simulink model "STEVE_Simulation"  (R2024b)
settings: Solver=ode4  StartTime=0.0  StopTime=60*1  FixedStep=0.001  RelTol=1e-3  EnableMultiTasking=on
values from neighbouring files (symbols this model uses):
  alphaValues = unique(data.Alpha)    [initialize_aeroData.m]    (also in initialize_parameters.m; lookup_data.mat = [0 2 4])
  CL_grid = nan(length(alphaValues), length(machValues))    [initialize_aeroData.m]    (also in initialize_parameters.m; lookup_data.mat = [0 0.430502365793 0.859237162153 0 0.432754592992 0.86375537)
  machValues = unique(data.Mach)    [initialize_aeroData.m]    (also in initialize_parameters.m; lookup_data.mat = [0.01 0.02 0.03 0.04 0.05 0.06 0.07 0.08 0.09 0.1 0.11 0.12 )
  max_thrust = 50    [initialize_parameters.m]
libraries: simulink x2, aerolibwind2 x1, aerolibatmos2 x1, simulink_extras x1, slpidlib x1, aerolibnav x1, aerolibasang x1, aerolibactuator x1
settings Model: ExtModeTrigDuration=2  Creator=jonno  LastModifiedBy=jonno
settings SolverCC: AutoInsertRateTranBlk=on
settings RTWCC: BuildConfiguration=Faster Runs

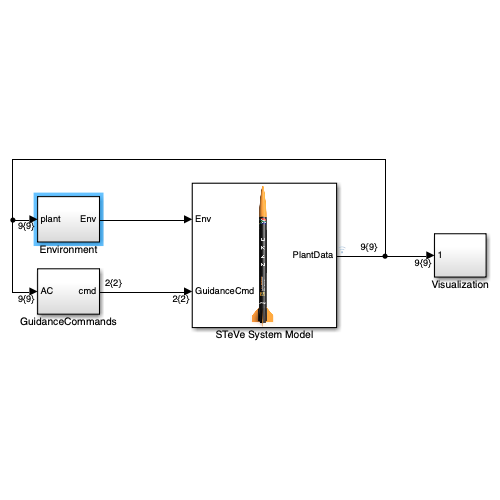
[thumbnail: Simulink's stored preview of the top-level diagram]
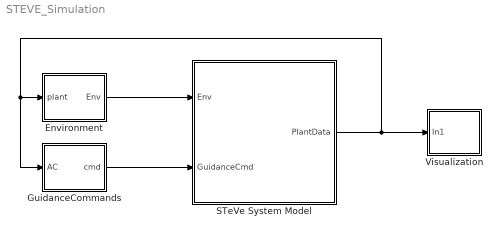
== system STEVE_Simulation ==
  Environment : Subsystem
  GuidanceCommands : Subsystem
  STeVe System Model : Subsystem
      mask Display: image('steve.png', [65 - (50 * (187 / 1041)), 0, 140 * (187 / 1041), 140])
  Visualization : Subsystem
  wires:
  GuidanceCommands/1(cmd) -> STeVe System Model/2(GuidanceCmd)
  Environment/1(Env) -> STeVe System Model/1(Env)
  STeVe System Model/1(PlantData) -> GuidanceCommands/1(AC), Environment/1(plant), Visualization/1(In1)

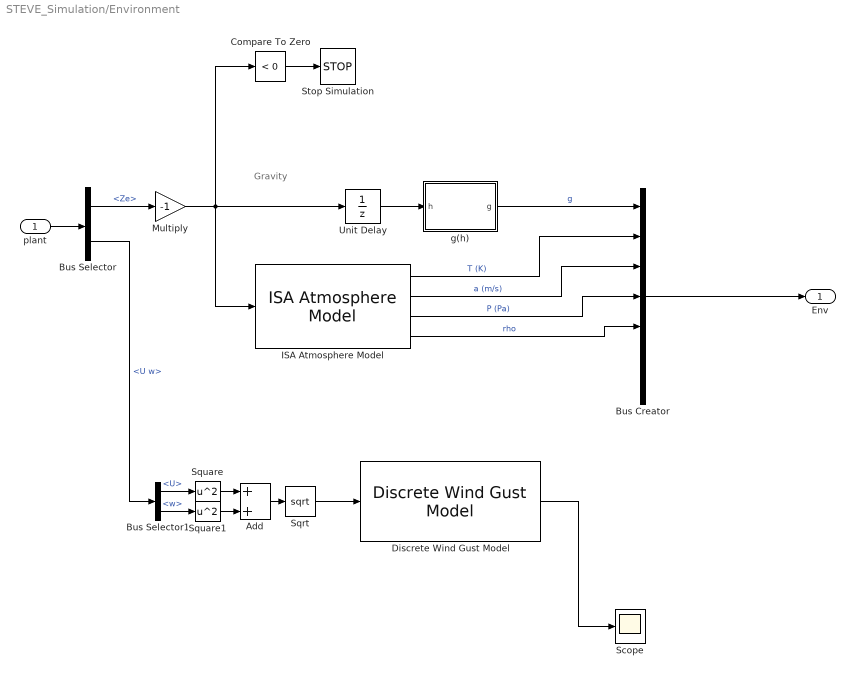
== system STEVE_Simulation/Environment ==
  note: Gravity
  plant : Inport
  Add : Sum
  Bus Creator : BusCreator  Inputs=7
  Bus Selector : BusSelector  OutputSignals=XeZe.Ze,U w
  Bus Selector1 : BusSelector  OutputSignals=U,w
  Compare To Zero : simulink/Logic and Bit Operations/Compare To Zero  relop=<  OutDataTypeStr=boolean
  Discrete Wind Gust Model : aerolibwind2/Discrete Wind Gust Model  units=Metric (MKS)  Gx=on  Gy=off  Gz=on  t_0=5  d_m=[120 120 80]  v_m=[3.5 3.5 3.0]
  ISA Atmosphere Model : aerolibatmos2/ISA Atmosphere Model  useExtended=on  action=Warning  custom=off  viscosityOut=off  g=9.80665  gamma=1.4  R=287.0531  L=0.0065  h_trop=11000  h_strat=20000  rho0=1.225  P0=101325  T0=288.15  h0=0  S=110.4  Tref=273.15  muref=1.716e-5
  Multiply : Gain  Gain=-1
  Scope : Scope
  Sqrt : Sqrt
  Square : Math  Operator=square
  Square1 : Math  Operator=square
  Stop Simulation : Stop
  Unit Delay : UnitDelay  SampleTime=-1  HasFrameUpgradeWarning=on
  g(h) : MATLAB Function  TreatAsAtomicUnit=on
  Env : Outport
  wires:
  g(h)/1(g) -> Bus Creator/1  "g"
  plant/1 -> Bus Selector/1
  Bus Selector/1 -> Multiply/1  "<Ze>"
  Bus Creator/1 -> Env/1
  Unit Delay/1 -> g(h)/1(h)
  Compare To Zero/1 -> Stop Simulation/1
  Multiply/1 -> ISA Atmosphere Model/1, Unit Delay/1, Compare To Zero/1
  ISA Atmosphere Model/1 -> Bus Creator/2  "T (K)"
  ISA Atmosphere Model/2 -> Bus Creator/3  "a (m/s)"
  ISA Atmosphere Model/3 -> Bus Creator/4  "P (Pa)"
  ISA Atmosphere Model/4 -> Bus Creator/5  "rho"
  ? -> Bus Creator/6  "u_wind_body"
  ? -> Bus Creator/7  "w_wind_body"
  Bus Selector/2 -> Bus Selector1/1  "<U w>"
  Bus Selector1/1 -> Square/1  "<U>"
  Bus Selector1/2 -> Square1/1  "<w>"
  Square1/1 -> Add/2
  Square/1 -> Add/1
  Add/1 -> Sqrt/1
  Sqrt/1 -> Discrete Wind Gust Model/1
  Discrete Wind Gust Model/1 -> Scope/1

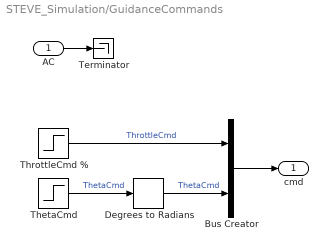
== system STEVE_Simulation/GuidanceCommands ==
  AC : Inport
  Bus Creator : BusCreator  Inputs=2
  Degrees to Radians : simulink_extras/Transformations/Degrees to Radians
  Terminator : Terminator
  ThetaCmd : Step  Before=90  After=170  SampleTime=0
  ThrottleCmd % : Step  Time=5  Before=100  After=0  SampleTime=0
  cmd : Outport
  wires:
  AC/1 -> Terminator/1
  ThrottleCmd %/1 -> Bus Creator/1  "ThrottleCmd"
  Bus Creator/1 -> cmd/1
  ThetaCmd/1 -> Degrees to Radians/1  "ThetaCmd"
  Degrees to Radians/1 -> Bus Creator/2  "ThetaCmd"

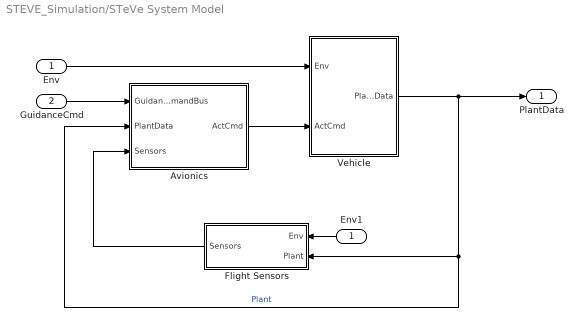
== system STEVE_Simulation/STeVe System Model ==
  Env : Inport
  GuidanceCmd : Inport  Port=2
  Avionics : Subsystem
  Env1 : InportShadow
  Flight Sensors : Subsystem
  Vehicle : Subsystem
  PlantData : Outport
  wires:
  Env/1 -> Vehicle/1(Env)
  Vehicle/1(PlantData) -> PlantData/1, Avionics/2(PlantData), Flight Sensors/2(Plant)  "Plant"
  Avionics/1(ActCmd) -> Vehicle/2(ActCmd)
  GuidanceCmd/1 -> Avionics/1(GuidanceCommandBus)
  Env1/1 -> Flight Sensors/1(Env)
  Flight Sensors/1(Sensors) -> Avionics/3(Sensors)

== system STEVE_Simulation/Visualization ==
  In1 : Inport
  Bus Selector : BusSelector  OutputSignals=XeZe
  Bus Selector1 : BusSelector  OutputSignals=Xe,Ze
  Compare To Zero : simulink/Logic and Bit Operations/Compare To Zero  relop=<  OutDataTypeStr=boolean
  Multiply : Gain  Gain=-1
  Stop Simulation : Stop
  XY Graph : Record  FileSettingsInternal="{\"entries\":[{\"content\":{\"excelSettings\":{\"content\":{},\"type\":\"Streamout.ExcelSettings\"}},\"type\":\"Streamout.FileSettingStorage\",\"uuid\":\"\"}],\"packageUris\":[\"http:\\/\\/schema.mathworks.com\\/mf0\\/streamout_blocks\\/R2020a\"],\"version\":\"1.0\"}"  Layout=[1 1]  SignalsInternal="{\"entries\":[{\"content\":{\"signals\":[{\"content\":{\"blockPath\":[],\"dimensions\":[1],\"domain\":\"\",\"lineColor\":\"#a2142f\",\"plots\":[ 1 ],\"port\":1,\"sid\":[\"\"],\"signalID\":1,\"signalName\":\"<Xe>\"},\"type\":\"RecordBlkView.Signal\",\"uuid\":\"\"},{\"content\":{\"blockPath\":[],\"dimensions\":[1],\"domain\":\"\",\"lineColor\":\"#139fff\",\"plots\":[ 1 ],\"port\":2,\"sid\":[\"\"],\"signalID\":2,\"signalName\":\"Multiply\"},\"type\":\"RecordBlkView.Signal\",\"uuid\":\"\"}]},\"type\":\"RecordBlkView.InputSignals\",\"uuid\":\"\"}],\"packageUris\":[\"http:\\/\\/schema.mathworks.com\\/mf0\\/streamout_blocks\\/R2020a\"],\"version\":\"1.0\"}"  VisualizationBindings="{\"xyplotplugin\":{\"info\":[{\"series\":[{\"bindingParametersList\":[{\"parameter\":\"X-Axis\",\"signalID\":1,\"signalName\":\"<Xe>\"},{\"parameter\":\"Y-Axis\",\"signalID\":2,\"signalName\":\"Multiply\"}],\"seriesID\":0}],\"subplotID\":1}]}}"  CompatibilityTag=XY
  wires:
  In1/1 -> Bus Selector/1
  Bus Selector/1 -> Bus Selector1/1  "<XeZe>"
  Bus Selector1/1 -> XY Graph/1  "<Xe>"
  Compare To Zero/1 -> Stop Simulation/1
  Bus Selector1/2 -> Multiply/1  "<Ze>"
  Multiply/1 -> Compare To Zero/1, XY Graph/2

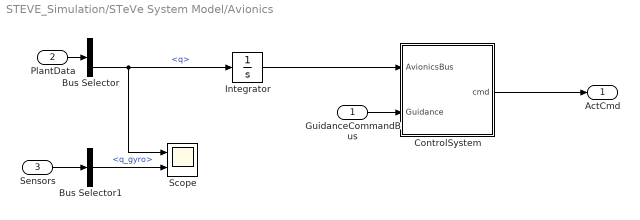
== system STEVE_Simulation/STeVe System Model/Avionics ==
  GuidanceCommandBus : Inport
  PlantData : Inport  Port=2
  Sensors : Inport  Port=3
  Bus Selector : BusSelector  OutputSignals=theta,q
  Bus Selector1 : BusSelector  OutputSignals=q_gyro
  ControlSystem : Subsystem
  Integrator : Integrator  InitialCondition=90*pi/180
  Scope : Scope  NumInputPorts=2
  ActCmd : Outport
  wires:
  PlantData/1 -> Bus Selector/1
  GuidanceCommandBus/1 -> ControlSystem/2(Guidance)
  ControlSystem/1(cmd) -> ActCmd/1
  Integrator/1 -> ControlSystem/1(AvionicsBus)
  Sensors/1 -> Bus Selector1/1
  Bus Selector/2 -> Scope/1, Integrator/1  "<q>"
  Bus Selector1/1 -> Scope/2  "<q_gyro>"

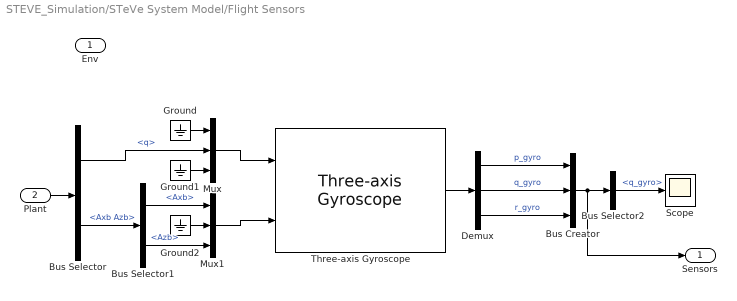
== system STEVE_Simulation/STeVe System Model/Flight Sensors ==
  Env : Inport
  Plant : Inport  Port=2
  Bus Creator : BusCreator  Inputs=3
  Bus Selector : BusSelector  OutputSignals=q,Axb Azb
  Bus Selector1 : BusSelector  OutputSignals=Axb,Azb
  Bus Selector2 : BusSelector  OutputSignals=q_gyro
  Demux : Demux  Outputs=3
  Ground : Ground
  Ground1 : Ground
  Ground2 : Ground
  Mux : Mux  Inputs=3
  Mux1 : Mux  Inputs=3
  Scope : Scope
  Three-axis Gyroscope : aerolibnav/Three-axis Gyroscope  dtype_g=on  w_g=190  z_g=0.707  g_sf_cc=[1 0 0; 0 1 0; 0 0 1]  g_bias=[0 0 0]  g_sen=[0 0 0]  g_Ts=0  g_rand=on  g_seeds=[23093 23094 23095]  g_pow=[0.0001 0.0001 0.0001]  g_sat="[-inf  -inf  -inf  inf inf inf]"
  Sensors : Outport
  wires:
  Plant/1 -> Bus Selector/1
  Mux/1 -> Three-axis Gyroscope/1
  Bus Selector/1 -> Mux/2  "<q>"
  Ground/1 -> Mux/1
  Ground1/1 -> Mux/3
  Mux1/1 -> Three-axis Gyroscope/2
  Bus Selector/2 -> Bus Selector1/1  "<Axb Azb>"
  Bus Selector1/1 -> Mux1/1  "<Axb>"
  Bus Selector1/2 -> Mux1/3  "<Azb>"
  Ground2/1 -> Mux1/2
  Three-axis Gyroscope/1 -> Demux/1
  Demux/1 -> Bus Creator/1  "p_gyro"
  Demux/2 -> Bus Creator/2  "q_gyro"
  Demux/3 -> Bus Creator/3  "r_gyro"
  Bus Creator/1 -> Sensors/1, Bus Selector2/1
  Bus Selector2/1 -> Scope/1  "<q_gyro>"

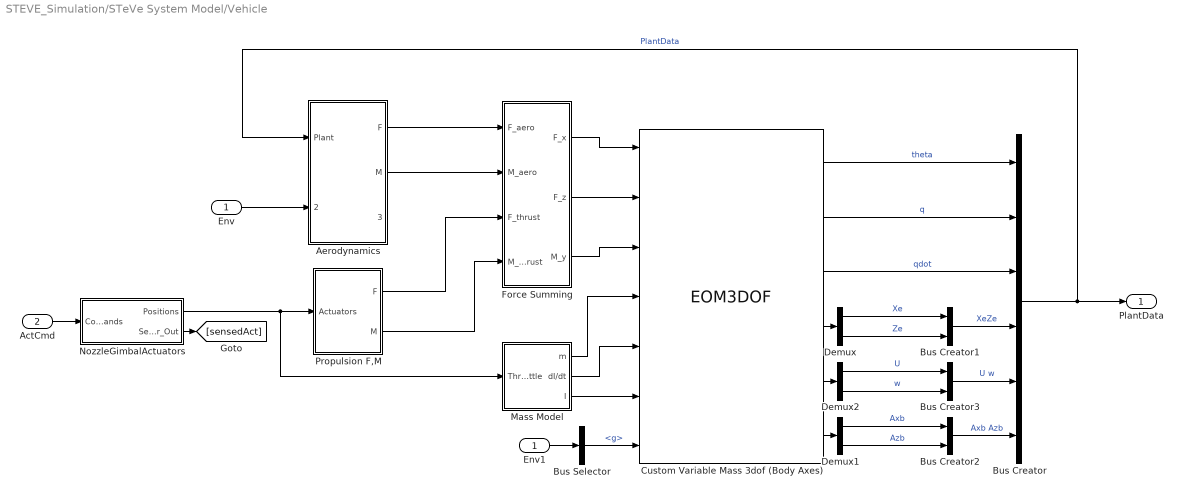
== system STEVE_Simulation/STeVe System Model/Vehicle ==
  Env : Inport
  ActCmd : Inport  Port=2
  Aerodynamics : Subsystem
  Bus Creator : BusCreator  Inputs=6
  Bus Creator1 : BusCreator  Inputs=2
  Bus Creator2 : BusCreator  Inputs=2
  Bus Creator3 : BusCreator  Inputs=2
  Bus Selector : BusSelector  OutputSignals=g
  Custom Variable Mass 3dof (Body Axes) : EOM3DOF  mtype=Custom Variable  v_ini=0  theta_ini=pi/2  g_in=External
  Demux : Demux  Outputs=2
  Demux1 : Demux  Outputs=2
  Demux2 : Demux  Outputs=2
  Env1 : InportShadow
  Force Summing : Subsystem
  Mass Model : Subsystem
  NozzleGimbalActuators : Subsystem
  Propulsion F,M : Subsystem
  PlantData : Outport
  wires:
  ActCmd/1 -> NozzleGimbalActuators/1(Commands)
  NozzleGimbalActuators/2(Sensor_Out) -> [sensedAct]
  NozzleGimbalActuators/1(Positions) -> Mass Model/1(Throttle), Propulsion F,M/1(Actuators)
  Force Summing/1(F_x) -> Custom Variable Mass 3dof (Body Axes)/1
  Force Summing/2(F_z) -> Custom Variable Mass 3dof (Body Axes)/2
  Aerodynamics/1(F) -> Force Summing/1(F_aero)
  Aerodynamics/2(M) -> Force Summing/2(M_aero)
  Propulsion F,M/1(F) -> Force Summing/3(F_thrust)
  Propulsion F,M/2(M) -> Force Summing/4(M_thrust)
  Force Summing/3(M_y) -> Custom Variable Mass 3dof (Body Axes)/3
  Mass Model/1(m) -> Custom Variable Mass 3dof (Body Axes)/4
  Mass Model/2(dI/dt) -> Custom Variable Mass 3dof (Body Axes)/5
  Mass Model/3(I) -> Custom Variable Mass 3dof (Body Axes)/6
  Custom Variable Mass 3dof (Body Axes)/1 -> Bus Creator/1  "theta"
  Custom Variable Mass 3dof (Body Axes)/2 -> Bus Creator/2  "q"
  Custom Variable Mass 3dof (Body Axes)/3 -> Bus Creator/3  "qdot"
  Bus Creator3/1 -> Bus Creator/5  "U w"
  Bus Creator2/1 -> Bus Creator/6  "Axb Azb"
  Bus Creator/1 -> Aerodynamics/1(Plant), PlantData/1  "PlantData"
  Bus Creator1/1 -> Bus Creator/4  "XeZe"
  Custom Variable Mass 3dof (Body Axes)/4 -> Demux/1
  Demux/1 -> Bus Creator1/1  "Xe"
  Demux/2 -> Bus Creator1/2  "Ze"
  Custom Variable Mass 3dof (Body Axes)/6 -> Demux1/1
  Demux1/1 -> Bus Creator2/1  "Axb"
  Demux1/2 -> Bus Creator2/2  "Azb"
  Custom Variable Mass 3dof (Body Axes)/5 -> Demux2/1
  Demux2/1 -> Bus Creator3/1  "U"
  Demux2/2 -> Bus Creator3/2  "w"
  Env/1 -> Aerodynamics/2(EnvData)
  Env1/1 -> Bus Selector/1
  Bus Selector/1 -> Custom Variable Mass 3dof (Body Axes)/7  "<g>"

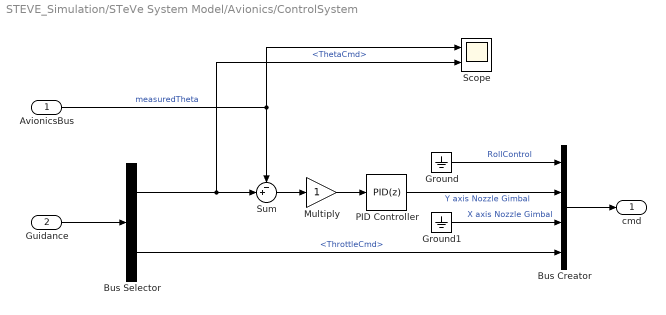
== system STEVE_Simulation/STeVe System Model/Avionics/ControlSystem ==
  AvionicsBus : Inport
  Guidance : Inport  Port=2
  Bus Creator : BusCreator  Inputs=4
  Bus Selector : BusSelector  OutputSignals=ThetaCmd,ThrottleCmd
  Ground : Ground
  Ground1 : Ground
  Multiply : Gain
  PID Controller : slpidlib/PID Controller  Controller=PID  Form=Parallel  TimeDomain=Discrete-time  UseExternalTs=off  SampleTime=-1  IntegratorMethod=Forward Euler  FilterMethod=Forward Euler  ControllerParametersSource=internal  P=1.9136005132319e-05  I=2.0107370615088e-06  UseKiTs=off  D=4.46649019604869e-05  UseExternalDerivativeSource=off  N=12.4167599537219  UseFilter=on  TunerSelectOption=Transfer Function Based (PID Tuner App)  InitialConditionSource=internal  InitialConditionForIntegrator=0  InitialConditionForFilter=0  DifferentiatorICPrevScaledInput=0  ExternalReset=none  TrackingMode=off  Kt=1  LimitOutput=off  SatLimitsSource=internal  UpperSaturationLimit=inf  LowerSaturationLimit=-inf  LinearizeAsGain=on  AntiWindupMode=none  Kb=1  LimitIntegrator=off  UpperIntegratorSaturationLimit=inf  LowerIntegratorSaturationLimit=-inf  POutMin=[]  POutMax=[]  IOutMin=[]  IOutMax=[]  DOutMin=[]  DOutMax=[]  NOutMin=[]  NOutMax=[]  SumOutMin=[]  SumOutMax=[]  SaturationOutMin=[]  SaturationOutMax=[]  PParamMin=[]  PParamMax=[]  IParamMin=[]  IParamMax=[]  DParamMin=[]  DParamMax=[]  NParamMin=[]  NParamMax=[]  KbParamMin=[]  KbParamMax=[]  KtParamMin=[]  KtParamMax=[]  KbOutMin=[]  KbOutMax=[]  KtOutMin=[]  KtOutMax=[]  IntegratorOutMin=[]  IntegratorOutMax=[]  FilterOutMin=[]  FilterOutMax=[]  SumI1OutMin=[]  SumI1OutMax=[]  SumI2OutMin=[]  SumI2OutMax=[]  SumI3OutMin=[]  SumI3OutMax=[]  SumI4OutMin=[]  SumI4OutMax=[]  SumDOutMin=[]  SumDOutMax=[]  DifferentiatorOutMin=[]  DifferentiatorOutMax=[]  FilterDiffOutCoefMin=[]  FilterDiffOutCoefMax=[]  ReciprocalOutMin=[]  ReciprocalOutMax=[]  SumDenOutMin=[]  SumDenOutMax=[]  SumNumOutMin=[]  SumNumOutMax=[]  DivideOutMin=[]  DivideOutMax=[]  UdiffTsProdOutMin=[]  UdiffTsProdOutMax=[]  NTsProdOutMin=[]  NTsProdOutMax=[]  UintegralTsProdOutMin=[]  UintegralTsProdOutMax=[]  UngainTsProdOutMin=[]  UngainTsProdOutMax=[]  ClampingZeroOutDataTypeStr=Inherit: Inherit via back propagation  ClampingZeroOutMin=[]  ClampingZeroOutMax=[]  FilterDenConstantOutDataTypeStr=Inherit: Inherit via back propagation  FilterDenConstantOutMin=[]  FilterDenConstantOutMax=[]  PCopyOutDataTypeStr=Inherit: Inherit via back propagation  PCopyOutMin=[]  PCopyOutMax=[]  NCopyOutDataTypeStr=Inherit: Inherit via back propagation  NCopyOutMin=[]  NCopyOutMax=[]  IntegratorContinuousStateAttributes=''  IntegratorStateMustResolveToSignalObject=off  IntegratorRTWStateStorageClass=Auto  FilterContinuousStateAttributes=''  FilterStateMustResolveToSignalObject=off  FilterRTWStateStorageClass=Auto  ParallelPVariant=InternalParameters  IdealPVariant=Disabled  IVariant=InternalParameters  DVariant=InternalParameters  IntegratorVariant=Discrete  SatVariant=Disabled  AWVariant=Passthrough  PCopyVariant=Disabled  TRVariant=Disabled  FdbkBlocksVariant=Forward  IdealPFdbkVariant=Disabled  SatFdbkVariant=Disabled  DerivativeFilterVariant=ForwardEulerFilter  NVariant=InternalParameters  NCopyVariant=Disabled  FilterICVariant=InternalICsFilter  IntegratorICVariant=InternalICs  ExternalResetVariant=Disabled  TRSumVariant=Passthrough  SumFdbkVariant=Disabled  SumVariant=Sum_PID  TsampFilterVariant=InternalTs  TsampNgainVariant=Passthrough  TsampIntegralVariant=Disabled_SignalSpec  ExternalSaturationOutDataTypeStr=Inherit: Same as second input  DerivativeSourceVariant=ErrorSignal  PreIntVariant=InternalPreInt
  Scope : Scope  NumInputPorts=2
  Sum : Sum  Inputs=-+|
  cmd : Outport
  wires:
  Bus Creator/1 -> cmd/1
  Ground/1 -> Bus Creator/1  "RollControl"
  PID Controller/1 -> Bus Creator/2  "Y axis Nozzle Gimbal"
  Ground1/1 -> Bus Creator/3  "X axis Nozzle Gimbal"
  Guidance/1 -> Bus Selector/1
  Bus Selector/2 -> Bus Creator/4  "<ThrottleCmd>"
  Bus Selector/1 -> Scope/2, Sum/2  "<ThetaCmd>"
  Sum/1 -> Multiply/1
  Multiply/1 -> PID Controller/1
  AvionicsBus/1 -> Sum/1, Scope/1  "measuredTheta"

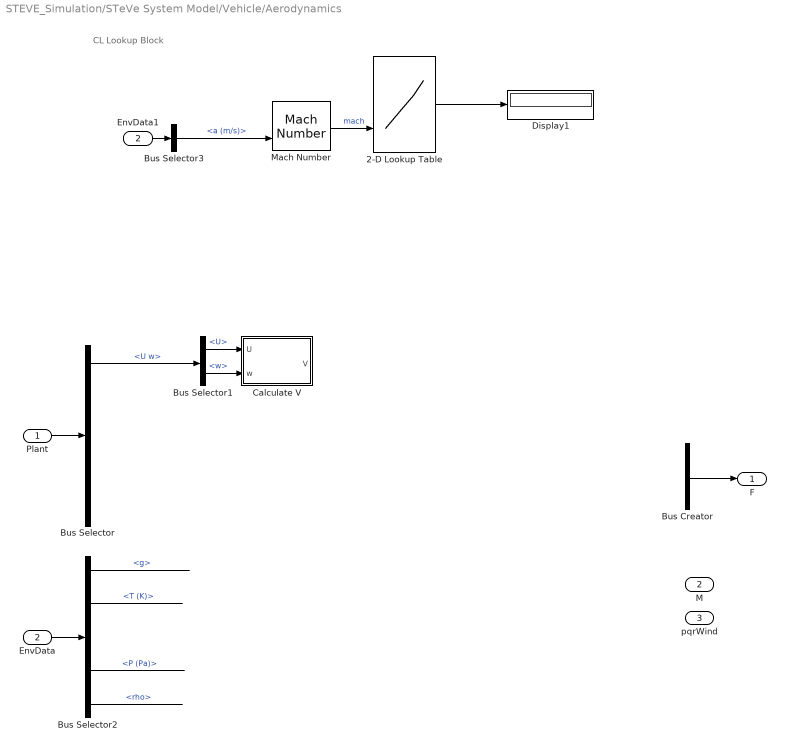
== system STEVE_Simulation/STeVe System Model/Vehicle/Aerodynamics ==
  note: CL Lookup Block
  Plant : Inport
  EnvData : Inport  Port=2
  2-D Lookup Table : Lookup_n-D  BreakpointsForDimension1=alphaValues  BreakpointsForDimension2=machValues  BeginIndexSearchUsingPreviousIndexResult=on  Table=CL_grid  InternalRulePriority=Speed  RndMeth=Simplest
      settings: InputPortMap=u0,u1
  Bus Creator : BusCreator  Inputs=2
  Bus Selector : BusSelector  OutputSignals=U w,theta,q,qdot,XeZe,U w,Axb Azb
  Bus Selector1 : BusSelector  OutputSignals=U,w
  Bus Selector2 : BusSelector  OutputSignals=g,T (K),a (m/s),P (Pa),rho
  Bus Selector3 : BusSelector  OutputSignals=a (m/s)
  Calculate V : MATLAB Function  TreatAsAtomicUnit=on
  Display1 : Display
  EnvData1 : InportShadow  Port=2
  Mach Number : aerolibasang/Mach Number
  F : Outport
  M : Outport  Port=2
  pqrWind : Outport  Port=3
  wires:
  Bus Creator/1 -> F/1
  ? -> Bus Creator/1  "Fa_x_b"
  Plant/1 -> Bus Selector/1
  EnvData/1 -> Bus Selector2/1
  Mach Number/1 -> 2-D Lookup Table/2  "mach"
  ? -> 2-D Lookup Table/1  "alpha"
  2-D Lookup Table/1 -> Display1/1
  ? -> Bus Creator/2  "Fa_z_b"
  ? -> pqrWind/1
  ? -> M/1  "Ma_y_b"
  Bus Selector1/1 -> Calculate V/1(U)  "<U>"
  Bus Selector1/2 -> Calculate V/2(w)  "<w>"
  Bus Selector/1 -> Bus Selector1/1  "<U w>"
  Bus Selector2/1 -> ?  "<g>"
  Bus Selector2/2 -> ?  "<T (K)>"
  Bus Selector2/4 -> ?  "<P (Pa)>"
  Bus Selector2/5 -> ?  "<rho>"
  EnvData1/1 -> Bus Selector3/1
  Bus Selector3/1 -> Mach Number/2  "<a (m/s)>"

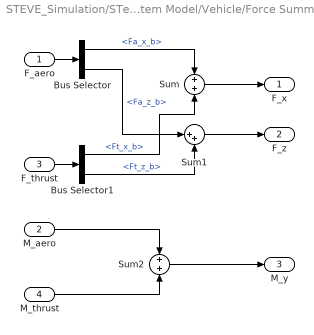
== system STEVE_Simulation/STeVe System Model/Vehicle/Force Summing ==
  F_aero : Inport
  M_aero : Inport  Port=2
  F_thrust : Inport  Port=3
  M_thrust : Inport  Port=4
  Bus Selector : BusSelector  OutputSignals=Fa_x_b,Fa_z_b
  Bus Selector1 : BusSelector  OutputSignals=Ft_x_b,Ft_z_b
  Sum : Sum
  Sum1 : Sum  Inputs=|++
  Sum2 : Sum
  F_x : Outport
  F_z : Outport  Port=2
  M_y : Outport  Port=3
  wires:
  F_aero/1 -> Bus Selector/1
  F_thrust/1 -> Bus Selector1/1
  Bus Selector/1 -> Sum/1  "<Fa_x_b>"
  Bus Selector1/1 -> Sum/2  "<Ft_x_b>"
  Sum/1 -> F_x/1
  Bus Selector1/2 -> Sum1/2  "<Ft_z_b>"
  Sum1/1 -> F_z/1
  Sum2/1 -> M_y/1
  M_aero/1 -> Sum2/1
  M_thrust/1 -> Sum2/2
  Bus Selector/2 -> Sum1/1  "<Fa_z_b>"

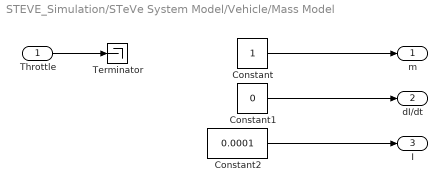
== system STEVE_Simulation/STeVe System Model/Vehicle/Mass Model ==
  Throttle : Inport
  Constant : Constant
  Constant1 : Constant  Value=0
  Constant2 : Constant  Value=0.0001
  Terminator : Terminator
  m : Outport
  dI/dt : Outport  Port=2
  I : Outport  Port=3
  wires:
  Constant/1 -> m/1
  Constant2/1 -> I/1
  Constant1/1 -> dI/dt/1
  Throttle/1 -> Terminator/1

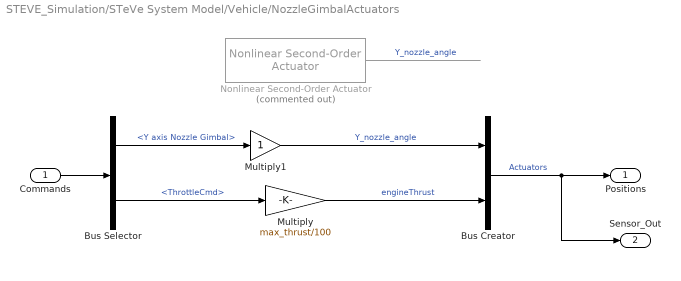
== system STEVE_Simulation/STeVe System Model/Vehicle/NozzleGimbalActuators ==
  Commands : Inport
  Bus Creator : BusCreator  Inputs=2
  Bus Selector : BusSelector  OutputSignals=Y axis Nozzle Gimbal,ThrottleCmd
  Multiply : Gain  Gain=max_thrust/100
  Multiply1 : Gain
  Nonlinear Second-Order Actuator : aerolibactuator/Nonlinear Second-Order Actuator  Commented=on  wn_fin=wn_act  z_fin=z_act  fin_max=maxdef_nozzle  fin_min=mindef_nozzle  fin_maxrate=rate_lim_nozzle  fin_act_0=0  fin_act_vel=0
  Positions : Outport
  Sensor_Out : Outport  Port=2
  wires:
  Commands/1 -> Bus Selector/1
  Bus Selector/1 -> Multiply1/1  "<Y axis Nozzle Gimbal>"
  Bus Creator/1 -> Positions/1, Sensor_Out/1  "Actuators"
  Bus Selector/2 -> Multiply/1  "<ThrottleCmd>"
  Multiply/1 -> Bus Creator/2  "engineThrust"
  Nonlinear Second-Order Actuator/1 -> ?  "Y_nozzle_angle"
  Multiply1/1 -> Bus Creator/1  "Y_nozzle_angle"

== system STEVE_Simulation/STeVe System Model/Vehicle/Propulsion F,M ==
  Actuators : Inport
  Bus Creator : BusCreator  Inputs=2
  Bus Selector : BusSelector  OutputSignals=engineThrust,Y_nozzle_angle
  MATLAB System : MATLABSystem  System=GimbalThrustModel  nozzleOffset=nozzle_moment_arm  SimulateUsing=Code generation
      mask Type: GimbalThrustModel
      mask Display:
      | disp('GimbalThrustModel');
      | port_label('input',1,'thrust');
      | port_label('input',2,'nozzle_angle');
      | port_label('output',1,'thrust_x');
      | port_label('output',2,'thrust_z');
      | port_label('output',3,'moment');
  F : Outport
  M : Outport  Port=2
  wires:
  Actuators/1 -> Bus Selector/1
  Bus Selector/2 -> MATLAB System/2  "<Y_nozzle_angle>"
  Bus Selector/1 -> MATLAB System/1  "<engineThrust>"
  MATLAB System/3 -> M/1  "M_y_b"
  MATLAB System/1 -> Bus Creator/1  "Ft_x_b"
  MATLAB System/2 -> Bus Creator/2  "Ft_z_b"
  Bus Creator/1 -> F/1

== matlab function STEVE_Simulation/Environment/g(h) ==
  data: h input; g output
function g = fcn(h)
G = 6.67430*10^(-11);
M = 5.9722*10^(24);
R_e = 6.371*10^(6);

g = (G * M)/(R_e + h)^2;

== matlab function STEVE_Simulation/STeVe System Model/Vehicle/Aerodynamics/Calculate V ==
  data: U input; V output; w input
function V = fcn(U, w)

V = (U^2 + w^2)^0.5;
